simulink model "eom-old"  (R2022b)
settings: Solver=FixedStepAuto  StartTime=0.0  StopTime=10.0  RelTol=1e-3
values from neighbouring files (symbols this model uses):
  theta_max = 1.0471975512    [constants.mat]
undefined symbols (not defined in the file or in its folder): alpha0, ic_alpha0
settings Model: Creator=KHods  LastModifiedBy=KHods
settings OptimizationCC: DefaultParameterBehavior=Inlined  UseDivisionForNetSlopeComputation=on  GainParamInheritBuiltInType=on  UseFloatMulNetSlope=on  InlineInvariantSignals=on  PassReuseOutputArgsThreshold=0  EfficientFloat2IntCast=on  OptimizeBlockOrder=speed  DifferentSizesBufferReuse=on
settings DebuggingCC: ParameterTunabilityLossMsg=error
settings HardwareCC: ProdLongLongMode=on  ProdHWDeviceType=AMD->x86-64 (Windows64)  TargetBitPerPointer=64  TargetBitPerSizeT=64  TargetBitPerPtrDiffT=64  TargetLongLongMode=on  TargetIntDivRoundTo=Zero  TargetEndianess=LittleEndian  TargetWordSize=64  TargetHWDeviceType=MATLAB Host  ProdEqTarget=off
settings SFSimCC: MATLABDynamicMemAlloc=off
settings RTWCC: Description=Rapid Simulation Target  SystemTargetFile=rsim.tlc  TemplateMakefile=rsim_default_tmf
settings CodeAppCC: ForceParamTrailComments=on  OperatorAnnotations=on
settings RSimTargetCC: TargetLangStandard=C99 (ISO)  OptimizeReductions=off

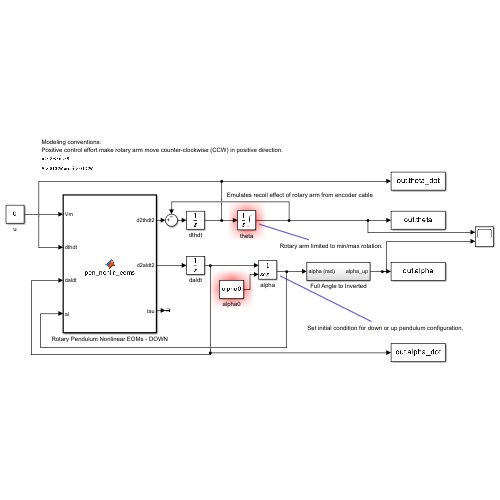
[thumbnail: Simulink's stored preview of the top-level diagram]
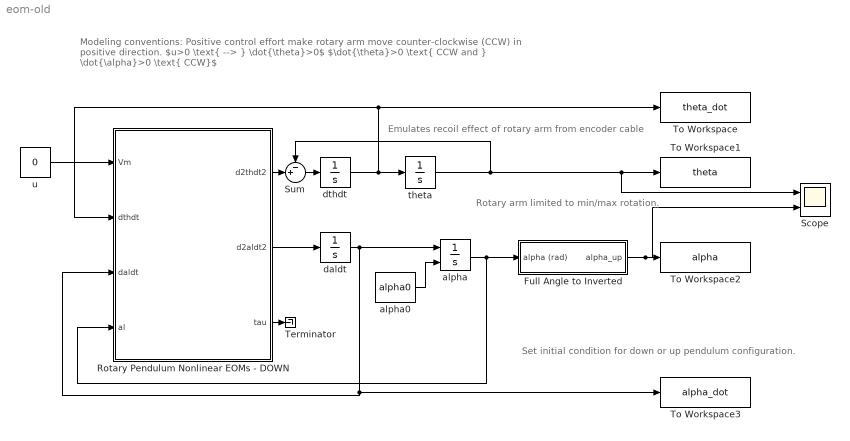
== system eom-old ==
  note: Set initial condition for down or up pendulum configuration.
  note: Rotary arm limited to min/max rotation.
  note: Emulates recoil effect of rotary arm from encoder cable
  note: Modeling conventions:
      | Positive control effort make rotary arm move counter-clockwise (CCW) in positive direction.
      | $u>0 \text{ --> } \dot{\theta}>0$
      | $\dot{\theta}>0 \text{ CCW and } \dot{\alpha}>0 \text{ CCW}$
  Full Angle to Inverted : Subsystem
  Rotary Pendulum Nonlinear EOMs - DOWN : MATLAB Function  TreatAsAtomicUnit=on
  Scope : Scope  NumInputPorts=2
  Sum : Sum  Inputs=-+|
  Terminator : Terminator
  To Workspace : ToWorkspace  VariableName=theta_dot  SampleTime=-1
      settings: Save2DSignal=2-D array (concatenate along first dimension)
  To Workspace1 : ToWorkspace  VariableName=theta  SampleTime=-1
      settings: Save2DSignal=2-D array (concatenate along first dimension)
  To Workspace2 : ToWorkspace  VariableName=alpha  SampleTime=-1
      settings: Save2DSignal=2-D array (concatenate along first dimension)
  To Workspace3 : ToWorkspace  VariableName=alpha_dot  SampleTime=-1
      settings: Save2DSignal=2-D array (concatenate along first dimension)
  alpha : Integrator  InitialConditionSource=external  InitialCondition=ic_alpha0  AbsoluteTolerance=1e-6
  alpha0 : Constant  Value=alpha0
  daldt : Integrator  AbsoluteTolerance=1e-6
  dthdt : Integrator  AbsoluteTolerance=1e-6
  theta : Integrator  LimitOutput=on  UpperSaturationLimit=theta_max  LowerSaturationLimit=-theta_max  AbsoluteTolerance=1e-6
  u : Constant  Value=0
  wires:
  theta/1 -> Scope/1, To Workspace1/1, Sum/1
  Rotary Pendulum Nonlinear EOMs - DOWN/1(d2thdt2) -> Sum/2
  Rotary Pendulum Nonlinear EOMs - DOWN/2(d2aldt2) -> daldt/1
  alpha0/1 -> alpha/2
  Full Angle to Inverted/1(alpha_up) -> Scope/2, To Workspace2/1
  dthdt/1 -> To Workspace/1, Rotary Pendulum Nonlinear EOMs - DOWN/2(dthdt), theta/1
  Sum/1 -> dthdt/1
  daldt/1 -> To Workspace3/1, Rotary Pendulum Nonlinear EOMs - DOWN/3(daldt), alpha/1
  Rotary Pendulum Nonlinear EOMs - DOWN/3(tau) -> Terminator/1
  alpha/1 -> Full Angle to Inverted/1(alpha (rad)), Rotary Pendulum Nonlinear EOMs - DOWN/4(al)
  u/1 -> Rotary Pendulum Nonlinear EOMs - DOWN/1(Vm)

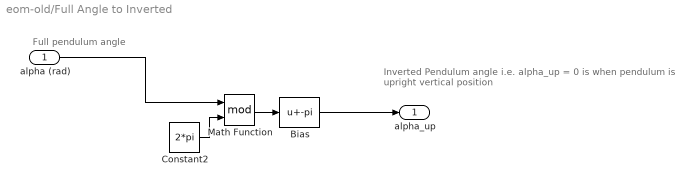
== system eom-old/Full Angle to Inverted ==
  note: Inverted Pendulum angle
      | i.e. alpha_up = 0 is when pendulum is upright vertical position
  note: Full pendulum angle
  alpha (rad) : Inport
  Bias : Bias  Bias=-pi  SaturateOnIntegerOverflow=off
  Constant2 : Constant  Value=2*pi
  Math Function : Math  Operator=mod  SignedPower=on
  alpha_up : Outport  VectorParamsAs1DForOutWhenUnconnected=off
  wires:
  Constant2/1 -> Math Function/2
  Bias/1 -> alpha_up/1
  alpha (rad)/1 -> Math Function/1
  Math Function/1 -> Bias/1

== matlab function eom-old/Rotary Pendulum Nonlinear EOMs - DOWN ==
  data: Vm input size=1; d2thdt2 output size=1; d2aldt2 output size=1; dthdt input size=1; daldt input size=1; al input size=1; tau output
function [d2thdt2,d2aldt2,tau] = pen_nonlin_eoms(Vm, dthdt, daldt, al)

% Resistance
Rm = 9.7; % nominal value = 8.4;
% Current-torque (N-m/A)
kt = 0.042;
% Back-emf constant (V-s/rad)
km = kt;
% Mass (kg)
mr = 0.095;
% Total length (m)
r = 0.085;
% Moment of inertia about pivot (kg-m^2)
Jr = mr*r^2/3;
% Equivalent Viscous Damping Coefficient (N-m-s/rad)
br = 1e-3; % damping tuned heuristically to match QUBE-Servo 2 response
% Mass (kg)
mp = 0.024;
% Total length (m)
Lp = 0.129;
% Pendulum center of mass (m)
l = Lp/2;
% Moment of inertia about pivot (kg-m^2)
Jp = mp*Lp^2/3;
% Equivalent Viscous Damping Coefficient (N-m-s/rad)
bp = 5e-5; % damping tuned heuristically to match QUBE-Sero 2 response
% Gravity Constant
g = 9.81;


% Convert voltage to torque input
tau = (Vm - km*dthdt)/Rm;
tau=kt*tau;
% Denominator
Jt = Jr*Jp + Jp^2*sin(al)^2 - mp^2*r^2*l^2*cos(al)^2;
% Nonlinear equations of motion for generic rotary pendulum (i.e. furuta)
% Terms from EOM solving
term1 = tau - br*dthdt + 2*Jp*sin(al)*cos(al)*dthdt*daldt + mp*r*l*sin(al)*daldt^2;
term2 = -bp*daldt - Jp*sin(al)*cos(al)*daldt^2 - mp*g*l*sin(al);
% Torque to rotary arm position)
d2thdt2 = 1/Jt*( Jp*term1 - mp*r*l*cos(al)*term2);
% Torque to pendulum angle position
d2aldt2 = 1/Jt*(-mp*r*l*cos(al)*term1 + (Jr+Jp*sin(al)^2)*term2);
